simulink model "EREV_1_Model_RL"  (R2025a)
settings: Solver=ode4  StartTime=0.0  StopTime=2474  FixedStep=0.05  MaxStep=0.01  RelTol=1e-3
values from neighbouring files (symbols this model uses):
  Af = 2.95    [EREV_RL_Parameters.m]
  bsfc_map = [ ... (first row only)    [EREV_RL_Parameters.m]
  Cd = 0.33    [EREV_RL_Parameters.m]
  eff_map_F = [ ... (first row only)    [EREV_RL_Parameters.m]
  eff_map_R = [ ... (first row only)    [EREV_RL_Parameters.m]
  eff_spd_F_rpm = [0    1000  2000  3000  4000  5000  6000  7000  8000  9000  10000 11000 12000]    [EREV_RL_Parameters.m]
  eff_spd_R_rpm = [0    1000  2000  3000  4000  5000  6000  7000  8000  9000  10000 11000 12000 13000 14000 15000]    [EREV_RL_Parameters.m]
  eff_trq_F = [0   26   53   79   106  132  158  185  211  238  264]    [EREV_RL_Parameters.m]
  eff_trq_R = [0   30   61   91   122  152  182  213  243  274  304]    [EREV_RL_Parameters.m]
  eng_speed_bsfc = [1000  1500  2000  2500  3000  3500  4000  4500  5000]    [EREV_RL_Parameters.m]
  eng_speed_rpm = [1000  1500  2000  2500  3000  3500  4000  4500  5000  5500  6000]    [EREV_RL_Parameters.m]
  eng_sweet_spot_speed = 2200    [EREV_RL_Parameters.m]
  eng_sweet_spot_torque = 180    [EREV_RL_Parameters.m]
  eng_torque_bsfc = [0  50  100  150  200  250]    [EREV_RL_Parameters.m]
  eng_torque_curve = [180   240   265   265   255   240   220   195   170   145   120]    [EREV_RL_Parameters.m]
  f_roll = 0.008    [EREV_RL_Parameters.m]
  g = 9.81    [EREV_RL_Parameters.m]
  G_final_F = 8.0    (= 8)    [EREV_RL_Parameters.m]
  G_final_R_1st = G_1st    (= 12)    [EREV_RL_Parameters.m]
  G_final_R_2nd = G_2nd    (= 7)    [EREV_RL_Parameters.m]
  h = 0.65    [EREV_RL_Parameters.m]
  M_veh = 2165    [EREV_RL_Parameters.m]
  Q_bat_Ah = 38.3    [EREV_RL_Parameters.m]
  Q_bat_kWh = 13.8    [EREV_RL_Parameters.m]
  R_int_base = 0.15    [EREV_RL_Parameters.m]
  R_multiplier = [3.0  2.0  1.5  1.2  1.1  1.0  1.0  1.1  1.2  1.8  2.5]    [EREV_RL_Parameters.m]
  r_tire = 0.369    [EREV_RL_Parameters.m]
  rho = 1.225    [EREV_RL_Parameters.m]
  shift_duration = 0.3    [EREV_RL_Parameters.m]
  SOC_init = 0.5    [EREV_RL_Parameters.m]
  SOC_R_table = [0.0  0.1  0.2  0.3  0.4  0.5  0.6  0.7  0.8  0.9  1.0]    [EREV_RL_Parameters.m]
  T_motor_F_curve = [264  264  264   264   264   250   230   210   195   180   168                      156  145   135   126   118   111   104    98    92    87    82    77    73    68]    [EREV_RL_Parameters.m]
  T_motor_R_curve = [304  304  304   304   304   304   295   280   265   250   235                      220  205   192   180   169   159   150   141   133   126   119                      113  107   101    96    91    86    82    78    74]    [EREV_RL_Parameters.m]
  T_motor_R_max = 304    [EREV_RL_Parameters.m]
  T_wheel_brake_max = 5000    [EREV_RL_Parameters.m]
  tau_m_F = 0.02    [EREV_RL_Parameters.m]
  tau_m_R = 0.02    [EREV_RL_Parameters.m]
  theta = 0    [EREV_RL_Parameters.m]
  torque_split_F_4wd = 0.4    [EREV_RL_Parameters.m]
  torque_split_R_4wd = 0.6    [EREV_RL_Parameters.m]
  V_downshift_kph = 30    [EREV_RL_Parameters.m]
  v_regen_min = 8    [EREV_RL_Parameters.m]
  V_upshift_kph = 35    [EREV_RL_Parameters.m]
  VOC_map = No_cell * VOC_cell    [EREV_RL_Parameters.m]
  VOC_SOC = [0    0.05  0.1   0.2   0.3   0.4   0.5   0.6   0.7   0.8   0.9   0.95  1.0]    [EREV_RL_Parameters.m]
  Vt_init = 374.4    [EREV_RL_Parameters.m]
  w_motor_F_rpm = [0    500  1000  1500  2000  2500  3000  3500  4000  4500  5000                    5500  6000  6500  7000  7500  8000  8500  9000  9500  10000 10500 11000 11500 12000]    [EREV_RL_Parameters.m]
  w_motor_R_rpm = [0    500  1000  1500  2000  2500  3000  3500  4000  4500  5000                    5500  6000  6500  7000  7500  8000  8500  9000  9500  10000 10500                   11000 11500 12000 12500 13000 13500 14000 14500 15000]    [EREV_RL_Parameters.m]
undefined symbols (not defined in the file or in its folder): T_brake_max, T_wheel_max_current
libraries: simulink x2, autolibshared x1, slpidlib x1, rllib x1
(part 2 of 2)

== system EREV_1_Model_RL/VCU/Level 2_TorqueCalculation ==
  note: T_wheel_brake
  Ap : Inport
  Bp : Inport  Port=2
  Gear_R : Inport  Port=3
  Gear_Ratio_Selection : Subsystem
  Pedal_to_Wheel_Torque : Subsystem
  To Workspace : ToWorkspace  VariableName=Gear_Actual  SaveFormat=Timeseries  SampleTime=-1
  To Workspace1 : ToWorkspace  VariableName=T_wheel_prop  SaveFormat=Timeseries  SampleTime=-1
  To Workspace2 : ToWorkspace  VariableName=T_wheel_brake  SaveFormat=Timeseries  SampleTime=-1
  To Workspace3 : ToWorkspace  VariableName=G_final_R  SaveFormat=Timeseries  SampleTime=-1
  T_wheel_prop : Outport
  T_wheel_brake : Outport  Port=2
  G_final_R : Outport  Port=3
  wires:
  Pedal_to_Wheel_Torque/2(T_wheel_brake) -> To Workspace2/1, T_wheel_brake/1
  Ap/1 -> Pedal_to_Wheel_Torque/1(Ap)
  Bp/1 -> Pedal_to_Wheel_Torque/2(Bp)
  Pedal_to_Wheel_Torque/1(T_wheel_prop) -> To Workspace1/1, T_wheel_prop/1
  Gear_Ratio_Selection/1(G_final_R) -> To Workspace/1, Pedal_to_Wheel_Torque/3(G_final_R), To Workspace3/1, G_final_R/1
  Gear_R/1 -> Gear_Ratio_Selection/1(RL_action)

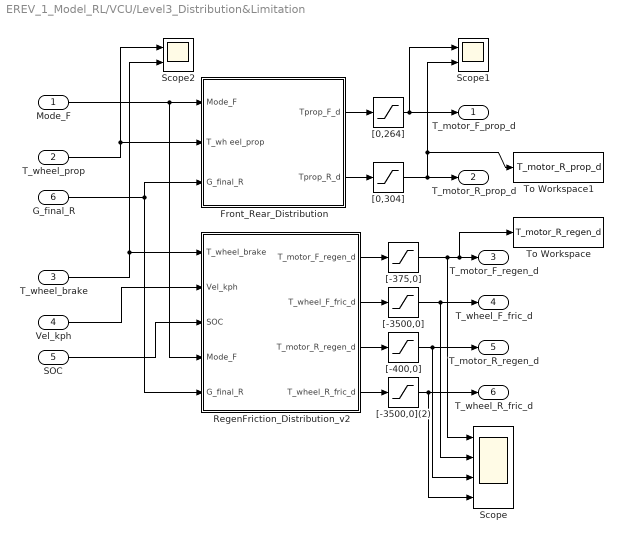
== system EREV_1_Model_RL/VCU/Level3_Distribution&Limitation ==
  Mode_F : Inport
  T_wheel_prop : Inport  Port=2
  T_wheel_brake : Inport  Port=3
  Vel_kph : Inport  Port=4
  SOC : Inport  Port=5
  G_final_R : Inport  Port=6
  Front_Rear_Distribution : Subsystem
  RegenFriction_Distribution_v2 : Subsystem
  Scope : Scope  NumInputPorts=4
      settings: ActiveDisplayYMinimum=-279.04024816839211  ActiveDisplayYMaximum=31.004472018710228  DataLoggingVariableName=ScopeData15
  Scope1 : Scope  NumInputPorts=2
      settings: DataLoggingVariableName=ScopeData16
  Scope2 : Scope  NumInputPorts=2
      settings: ActiveDisplayYMinimum=-1  ActiveDisplayYMaximum=1  DataLoggingVariableName=ScopeData17
  To Workspace : ToWorkspace  VariableName=T_motor_R_regen_d  SaveFormat=Timeseries  SampleTime=-1
  To Workspace1 : ToWorkspace  VariableName=T_motor_R_prop_d  SaveFormat=Timeseries  SampleTime=-1
  "[-3500,0]" : Saturate  UpperLimit=0  LowerLimit=-3500
  "[-3500,0](2)" : Saturate  UpperLimit=0  LowerLimit=-3500
  "[-375,0]" : Saturate  UpperLimit=0  LowerLimit=-375
  "[-400,0]" : Saturate  UpperLimit=0  LowerLimit=-400
  "[0,264]" : Saturate  UpperLimit=264  LowerLimit=0
  "[0,304]" : Saturate  UpperLimit=304  LowerLimit=0
  T_motor_F_prop_d : Outport
  T_motor_R_prop_d : Outport  Port=2
  T_motor_F_regen_d : Outport  Port=3
  T_wheel_F_fric_d : Outport  Port=4
  T_motor_R_regen_d : Outport  Port=5
  T_wheel_R_fric_d : Outport  Port=6
  wires:
  Mode_F/1 -> RegenFriction_Distribution_v2/4(Mode_F), Front_Rear_Distribution/1(Mode_F)
  T_wheel_prop/1 -> Scope2/1, Front_Rear_Distribution/2(T_wh eel_prop)
  Vel_kph/1 -> RegenFriction_Distribution_v2/2(Vel_kph)
  T_wheel_brake/1 -> Scope2/2, RegenFriction_Distribution_v2/1(T_wheel_brake)
  SOC/1 -> RegenFriction_Distribution_v2/3(SOC)
  "[0,264]"/1 -> Scope1/1, T_motor_F_prop_d/1
  RegenFriction_Distribution_v2/4(T_wheel_R_fric_d) -> "[-3500,0](2)"/1
  "[-3500,0](2)"/1 -> T_wheel_R_fric_d/1, Scope/4
  Front_Rear_Distribution/1(Tprop_F_d) -> "[0,264]"/1
  Front_Rear_Distribution/2(Tprop_R_d) -> "[0,304]"/1
  RegenFriction_Distribution_v2/1(T_motor_F_regen_d) -> "[-375,0]"/1
  RegenFriction_Distribution_v2/2(T_wheel_F_fric_d) -> "[-3500,0]"/1
  RegenFriction_Distribution_v2/3(T_motor_R_regen_d) -> "[-400,0]"/1
  "[-400,0]"/1 -> Scope/3, T_motor_R_regen_d/1
  "[-3500,0]"/1 -> Scope/2, T_wheel_F_fric_d/1
  "[0,304]"/1 -> To Workspace1/1, Scope1/2, T_motor_R_prop_d/1
  G_final_R/1 -> RegenFriction_Distribution_v2/5(G_final_R), Front_Rear_Distribution/3(G_final_R)
  "[-375,0]"/1 -> Scope/1, To Workspace/1, T_motor_F_regen_d/1

== system EREV_1_Model_RL/VCU/Level4_EngineControl ==
  Mode_F : Inport
  Engine_Command_Gen : Subsystem
  Engine_ONOFF_Logic : Subsystem
  Scope : Scope
      settings: ActiveDisplayYMinimum=-1  ActiveDisplayYMaximum=1  DataLoggingVariableName=ScopeData3
  Engine_Speed_cmd : Outport
  Engine_Torque_cmd : Outport  Port=2
  Engine_ON : Outport  Port=3
  tag scope: Engine_ON=global
  wires:
  Mode_F/1 -> Engine_ONOFF_Logic/1(Mode_F)
  Engine_Command_Gen/1(Engine_Speed_cmd) -> Engine_Speed_cmd/1
  Engine_Command_Gen/2(Engine_Torque_cmd) -> Scope/1, Engine_Torque_cmd/1
  Engine_ONOFF_Logic/1(Engine_ON) -> [Engine_ON], Engine_ON/1, Engine_Command_Gen/1(Engine_ON)

== system EREV_1_Model_RL/Vehicle/AerodynamicDrag ==
  v[m/s] : Inport
  Gain : Gain  Gain=Af
  Gain1 : Gain  Gain=rho
  Gain2 : Gain  Gain=Cd
  Gain3 : Gain  Gain=1/2
  Square : Math  Operator=square
  Faero : Outport
  wires:
  v[m/s]/1 -> Square/1
  Gain/1 -> Gain1/1
  Square/1 -> Gain/1
  Gain1/1 -> Gain2/1
  Gain2/1 -> Gain3/1
  Gain3/1 -> Faero/1  "Faero"

== system EREV_1_Model_RL/Vehicle/InclinedForce ==
  Constant : Constant  Value=theta
  Gain : Gain  Gain=M_veh*g
  Gain1 : Gain  Gain=pi/180
  Sin : Trigonometry
  Fslope[N] : Outport
  wires:
  Sin/1 -> Gain/1
  Gain/1 -> Fslope[N]/1  "Fslope"
  Constant/1 -> Gain1/1
  Gain1/1 -> Sin/1

== system EREV_1_Model_RL/Vehicle/RollingResistance ==
  v[m/s] : Inport
  Constant : Constant  Value=theta
  Cos : Trigonometry  Operator=cos
  Gain : Gain  Gain=M_veh*g
  Gain1 : Gain  Gain=f_roll
  Gain2 : Gain  Gain=pi/180
  Product : Product
  "[-1,1]" : Saturate  UpperLimit=1  LowerLimit=-1
  Froll[N] : Outport
  wires:
  v[m/s]/1 -> "[-1,1]"/1
  Cos/1 -> Gain/1
  Product/1 -> Froll[N]/1  "Froll"
  "[-1,1]"/1 -> Product/1
  Gain/1 -> Gain1/1
  Gain1/1 -> Product/2
  Gain2/1 -> Cos/1
  Constant/1 -> Gain2/1

== system EREV_1_Model_RL/Vehicle/Tire ==
  Tprop_out : Inport
  Tregen_out : Inport  Port=2
  Tfric_out : Inport  Port=3
  G_final_R : Inport  Port=4
  Gain1 : Gain  Gain=1/r_tire
  Sum : Sum  Inputs=+++
  Ftire : Outport
  wires:
  Gain1/1 -> Ftire/1  "Ftire"
  Tprop_out/1 -> Sum/1
  Tregen_out/1 -> Sum/2
  Sum/1 -> Gain1/1
  Tfric_out/1 -> Sum/3

== system EREV_1_Model_RL/VCU/Level 1_Mode&Gear Decision/Previous ==
  Gear_Selection : Subsystem
  Gear_Selection1 : Subsystem
  Mode_Selection : Subsystem
  SOC_Monitoring : Subsystem

== system EREV_1_Model_RL/VCU/Level 2_TorqueCalculation/Gear_Ratio_Selection ==
  RL_action : Inport
  Constant : Constant  Value=G_final_R_1st
  Constant1 : Constant  Value=G_final_R_2nd
  Constant2 : Constant  Value=0
  MATLAB Function : MATLAB Function  TreatAsAtomicUnit=on  SystemSampleTime=0.05
  Sampling Time (0.01s) : Constant  Value=0.05
  Switch : Switch  Criteria=u2 > Threshold  Threshold=0.5  SaturateOnIntegerOverflow=off  InputSameDT=off
  Switch1 : Switch  Criteria=u2 > Threshold  Threshold=1.5  SaturateOnIntegerOverflow=off  InputSameDT=off
  To Workspace : ToWorkspace  VariableName=Shift_In_Progress  SaveFormat=Timeseries  SampleTime=-1
  To Workspace1 : ToWorkspace  VariableName=Gear_R  SaveFormat=Timeseries  SampleTime=-1
  shift_duration (0.3s) : Constant  Value=shift_duration
  G_final_R : Outport
  Gear_R : Outport  Port=2
  tag scope: Gear_R=global, Gear_log=global, Shift_In_Progress=global
  wires:
  Constant/1 -> Switch1/3
  Constant1/1 -> Switch1/1
  Switch/1 -> G_final_R/1
  Sampling Time (0.01s)/1 -> MATLAB Function/2(Ts)
  shift_duration (0.3s)/1 -> MATLAB Function/3(shift_duration)
  MATLAB Function/2(Shift_In_Progress) -> To Workspace/1, [Shift_In_Progress]
  Constant2/1 -> Switch/3
  Switch1/1 -> Switch/1
  RL_action/1 -> MATLAB Function/1(Target_Gear)
  MATLAB Function/1(Gear_Actual) -> To Workspace1/1, [Gear_log], [Gear_R], Gear_R/1, Switch1/2, Switch/2

== system EREV_1_Model_RL/VCU/Level 2_TorqueCalculation/Pedal_to_Wheel_Torque ==
  Ap : Inport
  Bp : Inport  Port=2
  G_final_R : Inport  Port=3
  Gain1 : Gain  Gain=T_wheel_brake_max
  Gain2 : Gain  Gain=T_motor_R_max
  Product : Product
  T_wheel_prop : Outport
  T_wheel_brake : Outport  Port=2
  wires:
  Bp/1 -> Gain1/1
  Ap/1 -> Gain2/1
  Gain1/1 -> T_wheel_brake/1
  Product/1 -> T_wheel_prop/1
  Gain2/1 -> Product/2
  G_final_R/1 -> Product/1

== system EREV_1_Model_RL/VCU/Level3_Distribution&Limitation/Front_Rear_Distribution ==
  Mode_F : Inport
  T_wh eel_prop : Inport  Port=2
  G_final_R : Inport  Port=3
  Constant1 : Constant
  Constant2 : Constant  Value=0
  Divide1 : Product  Inputs=/*
  Divide2 : Product  Inputs=*/
  Gain : Gain  Gain=torque_split_R_4wd
  Gain1 : Gain  Gain=torque_split_F_4wd
  Gain2 : Gain  Gain=1/G_final_F
  Relational Operator : RelationalOperator  Operator===  OutDataTypeStr=boolean  RndMeth=Simplest  InputSameDT=off
  Switch : Switch  Criteria=u2 ~= 0  SaturateOnIntegerOverflow=off  InputSameDT=off
  Switch1 : Switch  Criteria=u2 ~= 0  SaturateOnIntegerOverflow=off  InputSameDT=off
  Tprop_F_d : Outport
  Tprop_R_d : Outport  Port=2
  wires:
  T_wh eel_prop/1 -> Gain/1, Gain1/1, Divide1/2  "Tprop_motor_d"
  Mode_F/1 -> Relational Operator/2
  Constant1/1 -> Relational Operator/1
  Relational Operator/1 -> Switch/2, Switch1/2
  Constant2/1 -> Switch/3
  Switch/1 -> Tprop_F_d/1
  Divide2/1 -> Switch1/1
  Gain/1 -> Divide2/1
  G_final_R/1 -> Divide2/2, Divide1/1
  Gain1/1 -> Gain2/1
  Gain2/1 -> Switch/1
  Divide1/1 -> Switch1/3
  Switch1/1 -> Tprop_R_d/1

== system EREV_1_Model_RL/VCU/Level3_Distribution&Limitation/RegenFriction_Distribution_v2 ==
  T_wheel_brake : Inport
  Vel_kph : Inport  Port=2
  SOC : Inport  Port=3
  Mode_F : Inport  Port=4
  G_final_R : Inport  Port=5
  Regen/Friction_Distribution Matlab Function : MATLAB Function  TreatAsAtomicUnit=on
  Scope : Scope  NumInputPorts=4
      settings: ActiveDisplayYMinimum=-1  ActiveDisplayYMaximum=1  DataLoggingVariableName=ScopeData13
  Scope1 : Scope  NumInputPorts=5
      settings: ActiveDisplayYMinimum=-5641.4095969862055  ActiveDisplayYMaximum=772.68637287585079  DataLoggingVariableName=ScopeData14
  T_motor_F_regen_d : Outport
  T_wheel_F_fric_d : Outport  Port=2
  T_motor_R_regen_d : Outport  Port=3
  T_wheel_R_fric_d : Outport  Port=4
  wires:
  G_final_R/1 -> Scope1/5, Regen/Friction_Distribution Matlab Function/5(G_final_R)
  Mode_F/1 -> Scope1/4, Regen/Friction_Distribution Matlab Function/4(Mode_F)
  SOC/1 -> Scope1/3, Regen/Friction_Distribution Matlab Function/3(SOC)
  Vel_kph/1 -> Regen/Friction_Distribution Matlab Function/2(Vel_kph), Scope1/2
  T_wheel_brake/1 -> Scope1/1, Regen/Friction_Distribution Matlab Function/1(T_wheel_brake)  "T_wheel_brake"
  Regen/Friction_Distribution Matlab Function/4(T_wheel_R_fric) -> Scope/4, T_wheel_R_fric_d/1
  Regen/Friction_Distribution Matlab Function/2(T_wheel_F_fric) -> Scope/2, T_wheel_F_fric_d/1
  Regen/Friction_Distribution Matlab Function/1(T_motor_F_regen) -> Scope/1, T_motor_F_regen_d/1
  Regen/Friction_Distribution Matlab Function/3(T_motor_R_regen) -> T_motor_R_regen_d/1, Scope/3

== system EREV_1_Model_RL/VCU/Level4_EngineControl/Engine_Command_Gen ==
  Engine_ON : Inport
  Constant : Constant  Value=eng_sweet_spot_torque
  Constant1 : Constant  Value=0
  Constant2 : Constant  Value=eng_sweet_spot_speed
  Constant3 : Constant  Value=0
  Switch : Switch  Criteria=u2 ~= 0  SaturateOnIntegerOverflow=off  InputSameDT=off
  Switch1 : Switch  Criteria=u2 > Threshold  SaturateOnIntegerOverflow=off  InputSameDT=off
  Engine_Speed_cmd : Outport
  Engine_Torque_cmd : Outport  Port=2
  wires:
  Engine_ON/1 -> Switch1/2, Switch/2
  Switch/1 -> Engine_Speed_cmd/1  "Engine_Speed_cmd"
  Switch1/1 -> Engine_Torque_cmd/1  "Engine_Torque_cmd"
  Constant1/1 -> Switch/3
  Constant3/1 -> Switch1/3
  Constant/1 -> Switch1/1
  Constant2/1 -> Switch/1

== system EREV_1_Model_RL/VCU/Level4_EngineControl/Engine_ONOFF_Logic ==
  Mode_F : Inport
  Constant : Constant  Value=2
  Equal : RelationalOperator  Operator===  OutDataTypeStr=boolean  RndMeth=Simplest  InputSameDT=off
  Engine_ON : Outport
  wires:
  Mode_F/1 -> Equal/1
  Constant/1 -> Equal/2
  Equal/1 -> Engine_ON/1

== system EREV_1_Model_RL/VCU/Level 1_Mode&Gear Decision/Previous/Gear_Selection ==
  Vel_kph : Inport
  Constant : Constant  Value=V_upshift_kph
  Constant1 : Constant  Value=V_downshift_kph
  Constant2 : Constant
  Constant3 : Constant  Value=2
  Constant4 : Constant  Value=2
  Constant5 : Constant
  Logical Operator : Logic  AllPortsSameDT=off  OutDataTypeStr=boolean
  Logical Operator1 : Logic  AllPortsSameDT=off  OutDataTypeStr=boolean
  Memory : Memory  InitialCondition=1
  Relational Operator : RelationalOperator  OutDataTypeStr=boolean  RndMeth=Simplest  InputSameDT=off
  Relational Operator1 : RelationalOperator  Operator===  OutDataTypeStr=boolean  RndMeth=Simplest  InputSameDT=off
  Relational Operator2 : RelationalOperator  Operator===  OutDataTypeStr=boolean  RndMeth=Simplest  InputSameDT=off
  Relational Operator3 : RelationalOperator  Operator=<=  OutDataTypeStr=boolean  RndMeth=Simplest  InputSameDT=off
  Switch : Switch  Criteria=u2 ~= 0  SaturateOnIntegerOverflow=off  InputSameDT=off
  Switch1 : Switch  Criteria=u2 ~= 0  SaturateOnIntegerOverflow=off  InputSameDT=off
  Gear_R : Outport
  wires:
  Vel_kph/1 -> Relational Operator/1, Relational Operator3/1
  Constant/1 -> Relational Operator/2
  Constant1/1 -> Relational Operator3/2
  Relational Operator/1 -> Logical Operator1/1  "upshift_speed_ok"
  Relational Operator3/1 -> Logical Operator/2  "downshift_speed_ok"
  Memory/1 -> Switch1/3, Relational Operator2/1, Relational Operator1/2
  Constant2/1 -> Relational Operator1/1
  Constant3/1 -> Relational Operator2/2
  Relational Operator1/1 -> Logical Operator1/2  "1st_gear"
  Relational Operator2/1 -> Logical Operator/1  "2nd_gear"
  Logical Operator1/1 -> Switch/2  "do_upshift"
  Logical Operator/1 -> Switch1/2  "do_downshift"
  Switch1/1 -> Switch/3
  Constant4/1 -> Switch/1
  Constant5/1 -> Switch1/1
  Switch/1 -> Memory/1, Gear_R/1

== system EREV_1_Model_RL/VCU/Level 1_Mode&Gear Decision/Previous/Gear_Selection1 ==
  Vel_kph : Inport
  VCU_mode : Inport  Port=2
  Constant : Constant  Value=V_upshift_kph
  Constant1 : Constant  Value=V_downshift_kph
  MATLAB Function : MATLAB Function  TreatAsAtomicUnit=on  SystemSampleTime=0.01
  Gear_R : Outport
  wires:
  VCU_mode/1 -> MATLAB Function/1(VCU_mode)
  MATLAB Function/1(Gear_R) -> Gear_R/1
  Constant1/1 -> MATLAB Function/4(V_downshift_kph)
  Constant/1 -> MATLAB Function/3(V_upshift_kph)
  Vel_kph/1 -> MATLAB Function/2(Vel_kph)

== system EREV_1_Model_RL/VCU/Level 1_Mode&Gear Decision/Previous/Mode_Selection ==
  sys_mode : Inport
  Ap : Inport  Port=2
  Constant1 : Constant  Value=0
  Constant2 : Constant  Value=2
  Constant3 : Constant
  Constant4 : Constant  Value=0.5
  Logical Operator : Logic  AllPortsSameDT=off  OutDataTypeStr=boolean
  Relational Operator : RelationalOperator  Operator===  OutDataTypeStr=boolean  RndMeth=Simplest  InputSameDT=off
  Relational Operator1 : RelationalOperator  Operator===  OutDataTypeStr=boolean  RndMeth=Simplest  InputSameDT=off
  Relational Operator2 : RelationalOperator  Operator=>  OutDataTypeStr=boolean  RndMeth=Simplest  InputSameDT=off
  Switch : Switch  Criteria=u2 ~= 0  SaturateOnIntegerOverflow=off  InputSameDT=off
  Switch1 : Switch  Criteria=u2 ~= 0  SaturateOnIntegerOverflow=off  InputSameDT=off
  Mode_F : Outport
  wires:
  Ap/1 -> Relational Operator2/1
  sys_mode/1 -> Relational Operator/1, Relational Operator1/2
  Constant2/1 -> Relational Operator1/1, Switch1/1  "Mode_F=2(Generator)"
  Constant1/1 -> Switch/3, Relational Operator/2  "Mode_F=0 (2WD Disconnect)"
  Relational Operator/1 -> Logical Operator/1  "EV_mode"
  Relational Operator1/1 -> Switch1/2  "charge_mode"
  Switch/1 -> Switch1/3
  Logical Operator/1 -> Switch/2
  Constant3/1 -> Switch/1  "Mode_F=1 (4WD Motor)"
  Constant4/1 -> Relational Operator2/2
  Relational Operator2/1 -> Logical Operator/2  "Ap_high"
  Switch1/1 -> Mode_F/1  "Mode_Front"

== system EREV_1_Model_RL/VCU/Level 1_Mode&Gear Decision/Previous/SOC_Monitoring ==
  SOC : Inport
  Constant : Constant  Value=2
  Constant1 : Constant  Value=0
  Memory : Memory
  Switch : Switch  Criteria=u2 > Threshold  Threshold=0.3  SaturateOnIntegerOverflow=off  InputSameDT=off
  Switch1 : Switch  Threshold=0.4  SaturateOnIntegerOverflow=off  InputSameDT=off
  sys_mode : Outport
  wires:
  SOC/1 -> Switch1/2, Switch/2
  Constant/1 -> Switch/3
  Constant1/1 -> Switch1/1
  Memory/1 -> Switch/1
  Switch/1 -> Switch1/3
  Switch1/1 -> Memory/1, sys_mode/1

== matlab function EREV_1_Model_RL/Trash/RegenFriction_Distribution/MATLAB Function1 ==
  data: Tbrake_motor_d input; Tregen_d output; SOC input; Vel_kph input; Tfric_d output
function [Tregen_d, Tfric_d] = RegenFriction_Distribution(Tbrake_motor_d, SOC, Vel_kph)
    regen_enable = (Vel_kph > 10) && (SOC < 0.9);
    
    if regen_enable
        Tregen_max = 203;
        if SOC > 0.8
            Tregen_max = Tregen_max * 0.5;
        end
        
        Tregen_d = min(Tbrake_motor_d, Tregen_max);
        Tfric_d = Tbrake_motor_d - Tregen_d;
    else
        Tregen_d = 0;
        Tfric_d = Tbrake_motor_d;
    end
end

== matlab function EREV_1_Model_RL/Trash/Mode_Selection/MATLAB Function ==
  data: sys_mode input; Mode_F output; Ap input
function Mode_F = Mode_Selection(sys_mode, Ap)
    switch sys_mode
        case 0  % EV 모드
            if Ap > 50  % 페달 기준 ✅
                Mode_F = 1;  % 4WD
            else
                Mode_F = 0;  % 2WD
            end
        case 1  % Hybrid
            Mode_F = 1;
        case 2  % Charge
            Mode_F = 2;
    end
end

== matlab function EREV_1_Model_RL/VCU/Level3_Distribution&Limitation/RegenFriction_Distribution_v2/Regen//Friction_Distribution Matlab Function ==
  data: T_wheel_brake input; T_motor_F_regen output; Vel_kph input; SOC input; Mode_F input; G_final_R input; T_wheel_F_fric output; T_motor_R_regen output; T_wheel_R_fric output
function [T_motor_F_regen, T_wheel_F_fric, T_motor_R_regen, T_wheel_R_fric] = ...
    RegenFrictionDistribution(T_wheel_brake, Vel_kph, SOC, Mode_F, G_final_R)
%#codegen
% ========================================================================
% EREV Regenerative & Friction Braking Distribution (수정 버전)
% ========================================================================

%% 파라미터
G_final_F = 7.94;
T_motor_F_max = 264;  % Nm (정격 최대 토크)
T_motor_R_max = 304;  % Nm
P_motor_F_max = 67000;  % W
P_motor_R_max = 91000;  % W

regen_ratio_max = 0.8;  % 정격 토크의 80%까지 회생
brake_regen_ratio_max = 0.7;  % 총 제동의 70%까지 회생 허용

v_regen_min = 8;    % km/h
v_regen_full = 15;  % km/h
regen_max_SOC = 0.9;

torque_split_F_4wd = 0.4;
torque_split_R_4wd = 0.6;

%% Step 1: Mode에 따른 전후륜 토크 분배
if Mode_F == 0
    torque_split_F = 0.0;
    torque_split_R = 1.0;
elseif Mode_F == 1
    torque_split_F = torque_split_F_4wd;
    torque_split_R = torque_split_R_4wd;
else
    torque_split_F = 0.0;
    torque_split_R = 1.0;
end

% 전후륜 휠 제동 토크 (음수)
T_wheel_brake_F = T_wheel_brake * torque_split_F;
T_wheel_brake_R = T_wheel_brake * torque_split_R;

%% Step 2: 회생제동 가능 여부 (속도, SOC 기반)
if Vel_kph < v_regen_min
    vel_factor = 0.0;
elseif Vel_kph < v_regen_full
    vel_factor = (Vel_kph - v_regen_min) / (v_regen_full - v_regen_min);
else
    vel_factor = 1.0;
end

if SOC >= regen_max_SOC
    soc_factor = 0.0;
else
    soc_factor = 1.0;
end

regen_available = vel_factor * soc_factor;

%% Step 3: RPM 계산 및 파워 제한
r_tire = 0.369;  % m
w_wheel = Vel_kph / 3.6 / r_tire;  % rad/s

w_motor_F = w_wheel * G_final_F;
w_motor_R = w_wheel * G_final_R;

%% Step 4: 모터별 회생 최대 토크 계산

% === 전륜 ===
% (1) 정격 토크 제한
T_motor_F_limit_rated = -T_motor_F_max * regen_ratio_max;  % -211 Nm

% (2) 파워 제한
if w_motor_F > 0.1
    T_motor_F_limit_power = -P_motor_F_max / w_motor_F;
else
    T_motor_F_limit_power = T_motor_F_limit_rated;
end

% (3) 최종 한계 = 둘 중 작은 것 (절댓값 기준)
T_motor_F_max_regen = max(T_motor_F_limit_rated, T_motor_F_limit_power);

% === 후륜 ===
T_motor_R_limit_rated = -T_motor_R_max * regen_ratio_max;  % -243 Nm

if w_motor_R > 0.1
    T_motor_R_limit_power = -P_motor_R_max / w_motor_R;
else
    T_motor_R_limit_power = T_motor_R_limit_rated;
end

T_motor_R_max_regen = max(T_motor_R_limit_rated, T_motor_R_limit_power);

%% Step 5: 요구 모터 토크 계산
% 휠 제동 토크 → 모터 토크 변환
T_motor_brake_F_request = T_wheel_brake_F / G_final_F;
T_motor_brake_R_request = T_wheel_brake_R / G_final_R;

%% Step 6: 회생 제동 결정

% (1) 회생 가능 토크 (속도/SOC 고려)
T_motor_F_regen_possible = T_motor_F_max_regen * regen_available;
T_motor_R_regen_possible = T_motor_R_max_regen * regen_available;

% (2) 70% 제한 적용 (요구의 70%까지만)
T_motor_F_regen_70pct = T_motor_brake_F_request * brake_regen_ratio_max;
T_motor_R_regen_70pct = T_motor_brake_R_request * brake_regen_ratio_max;

% (3) 최종 회생 토크 = min(가능, 70%제한, 요구) (절댓값 기준)
% max()는 음수에서 절댓값이 작은 것 선택
T_motor_F_regen = max([T_motor_F_regen_possible, T_motor_F_regen_70pct, T_motor_brake_F_request]);
T_motor_R_regen = max([T_motor_R_regen_possible, T_motor_R_regen_70pct, T_motor_brake_R_request]);

%% Step 7: 마찰 제동 보충
% 회생으로 만드는 휠 토크
T_wheel_F_regen = T_motor_F_regen * G_final_F;
T_wheel_R_regen = T_motor_R_regen * G_final_R;

% 부족분을 마찰 제동으로
T_wheel_F_fric = T_wheel_brake_F - T_wheel_F_regen;
T_wheel_R_fric = T_wheel_brake_R - T_wheel_R_regen;

% 음수 방향으로만 (제동)
T_wheel_F_fric = min(T_wheel_F_fric, 0.0);
T_wheel_R_fric = min(T_wheel_R_fric, 0.0);

%% Step 8: 예외 처리
if regen_available < 0.01
    % 회생 불가능 → 전부 마찰 제동
    T_motor_F_regen = 0.0;
    T_motor_R_regen = 0.0;
    T_wheel_F_fric = T_wheel_brake_F;
    T_wheel_R_fric = T_wheel_brake_R;
end

end

== matlab function EREV_1_Model_RL/Trash/Gear_Selection/MATLAB Function ==
  data: Vel_kph input; Gear_R output; Ap input
function Gear_R = Gear_Selection(Vel_kph, Ap)
    persistent prev_gear;
    if isempty(prev_gear)
        prev_gear = 1;
    end
    
    if Vel_kph >= 60 && prev_gear == 1
        Gear_R = 2;
    elseif Vel_kph <= 55 && prev_gear == 2
        Gear_R = 1;
    elseif Ap > 80 && Vel_kph < 80 && prev_gear == 2
        Gear_R = 1;  % 킥다운
    else
        Gear_R = prev_gear;
    end
    
    prev_gear = Gear_R;
end

== matlab function EREV_1_Model_RL/Trash/Front_Rear_Distribution/MATLAB Function ==
  data: Tprop_motor_d input; Tprop_F_d output; Mode_F input; G_final_R input; Tprop_R_d output
function [Tprop_F_d, Tprop_R_d] = FrontRear_Distribution(Tprop_motor_d, Mode_F, G_final_R)
    G_final_F = 8;
    
    if Mode_F == 1  % 4WD
        % 전후륜 50:50 분배
        T_wheel_total = Tprop_motor_d * G_final_R;
        T_wheel_F = T_wheel_total * 0.5;
        T_wheel_R = T_wheel_total * 0.5;
        
        Tprop_F_d = T_wheel_F / G_final_F;
        Tprop_R_d = T_wheel_R / G_final_R;
    else  % 2WD
        Tprop_F_d = 0;
        Tprop_R_d = Tprop_motor_d;
    end
end

== matlab function EREV_1_Model_RL/VCU/Level 2_TorqueCalculation/Gear_Ratio_Selection/MATLAB Function ==
  data: Target_Gear input; Gear_Actual output; Ts input; shift_duration input; Shift_In_Progress output
function [Gear_Actual, Shift_In_Progress] = ShiftDurationLogic(Target_Gear, Ts, shift_duration)
    % Target_Gear: RL이나 Decoder에서 들어오는 목표 기어 (1 또는 2)
    % Ts: 시뮬레이션 샘플 타임 (예: 0.01s)
    % shift_duration: 변속 소요 시간 (예: 0.3s)
    
    persistent current_gear latched_target_gear shift_timer is_shifting
    
    % 초기화 (최초 실행 시)
    if isempty(current_gear)
        current_gear = 1;          % 초기 기어는 1단으로 가정
        latched_target_gear = 1;   % 목표 기어 초기화
        shift_timer = 0;
        is_shifting = false;
    end
    
    %% 1. 변속 트리거 로직 (Toggle -> Target Comparison)
    % 현재 변속 중이 아니고, 목표 기어가 현재 기어와 다르면 변속 시작
    if (Target_Gear ~= current_gear) && ~is_shifting
        is_shifting = true;
        shift_timer = 0;
        latched_target_gear = Target_Gear; % 목표 기어 확정(Latch)
    end
    
    %% 2. 변속 진행 로직 (시간 지연)
    if is_shifting
        shift_timer = shift_timer + Ts;
        
        % 변속 시간이 지났으면 기어 변경 완료
        if shift_timer >= shift_duration
            current_gear = latched_target_gear; % 기어 변경
            is_shifting = false;
            shift_timer = 0;
        end
    end
    
    %% 3. 최종 출력
    if is_shifting
        Gear_Actual = 0; % 변속 중에는 중립(0) -> 동력 끊김 구현
    else
        Gear_Actual = current_gear; % 변속 완료 시 해당 기어 출력
    end
    
    Shift_In_Progress = is_shifting;
end

== matlab function EREV_1_Model_RL/Trash/Motor_Limit_Check/MATLAB Function ==
  data: Tprop_motor_d input; Tprop_limited output; w_motor_R input
% w_motor_R 입력이 있을 때만 사용
function Tprop_limited = Motor_Limit_Check(Tprop_motor_d, w_motor_R)
    % 속도-토크 특성
    w_spd = [0 300 419 524 628 733 838 943 1047 1152 1257 1361] * (pi/30);
    T_max = [203 203 193 156 129 111 98 85 79 72 65 60];
    
    % 현재 속도에서 최대 토크
    T_motor_max = interp1(w_spd, T_max, w_motor_R, 'linear', 60);
    
    % 제한
    Tprop_limited = min(Tprop_motor_d, T_motor_max);
end

== matlab function EREV_1_Model_RL/VCU/Level 1_Mode&Gear Decision/MATLAB Function ==
  data: RL_Action input; Target_Gear output; SOC input; Mode_F output; Ap input
function [Target_Gear, Mode_F] = Action_Decoder(RL_Action, SOC, Ap)
    % Action Decoder (RL 중심)
    
    %% 1. RL 의도 해석
    % 기어: 1,3은 1단 / 2,4는 2단
    if (RL_Action == 1) || (RL_Action == 3)
        Target_Gear = 1;
    else
        Target_Gear = 2;
    end
    
    % 발전 요청: 3,4는 발전
    if (RL_Action == 3) || (RL_Action == 4)
        req_gen = 1;
    else
        req_gen = 0;
    end
    
    %% 2. 최소 안전 로직 (SOC 하한만)
    if SOC < 0.25
        Mode_F = 2;     % 강제 발전 (위급 상황)
    elseif req_gen == 1
        Mode_F = 2;     % RL 요청: 발전
    elseif Ap > 0.5
        Mode_F = 1;     % 급가속: 4WD
    else
        Mode_F = 0;     % 일반 주행: 2WD
    end
end

== matlab function EREV_1_Model_RL/VCU/Level 1_Mode&Gear Decision/Previous/Gear_Selection1/MATLAB Function ==
  settings: updateMethod=DISCRETE
  data: VCU_mode input; Gear_R output; Vel_kph input; V_upshift_kph input; V_downshift_kph input
function Gear_R = GearSelection(VCU_mode, Vel_kph, V_upshift_kph, V_downshift_kph)
    % VCU_mode: 1=2단변속, 2=1단고정, 3=2단고정
    % Vel_kph: 차량 속도
    % V_upshift_kph: 업시프트 속도 (35)
    % V_downshift_kph: 다운시프트 속도 (30)
    
    persistent current_gear
    
    % 초기화
    if isempty(current_gear)
        current_gear = 1;
    end
    
    % VCU 모드에 따른 기어 선택
    if VCU_mode == 2
        % 1단 고정
        Gear_R = 1;
        current_gear = 1;  % persistent 변수도 업데이트
        
    elseif VCU_mode == 3
        % 2단 고정
        Gear_R = 2;
        current_gear = 2;
        
    else
        % VCU_mode == 1: 2단 변속 (기존 로직)
        
        % 업시프트 (1단 → 2단)
        if current_gear == 1 && Vel_kph >= V_upshift_kph
            current_gear = 2;
        end
        
        % 다운시프트 (2단 → 1단)
        if current_gear == 2 && Vel_kph <= V_downshift_kph
            current_gear = 1;
        end
        
        Gear_R = current_gear;
    end
end

== matlab function EREV_1_Model_RL/Trash/Engine_Command_Gen/MATLAB Function ==
  data: Engien_ON input; Engine_Speed_cmd output; Engine_Torque_cmd output
function [Engine_Speed_cmd, Engine_Torque_cmd] =Engine_Command_Gen(Engien_ON)

if Engine_ON
    Engine_Speed_cmd=2000;
    Engine_Torque_cmd=150;
else
    Engine_Speed_cmd=0;
    Engine_Torque_cmd=0;
end
